simulink model "stimfun"  (R2023a)
settings: Solver=VariableStepAuto  StartTime=0.0  StopTime=10.0  RelTol=1e-3
libraries: simulink x1
settings Model: Creator=s202421  LastModifiedBy=s202421

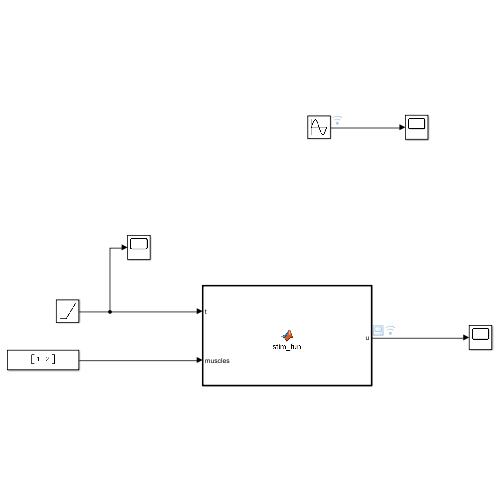
[thumbnail: Simulink's stored preview of the top-level diagram]
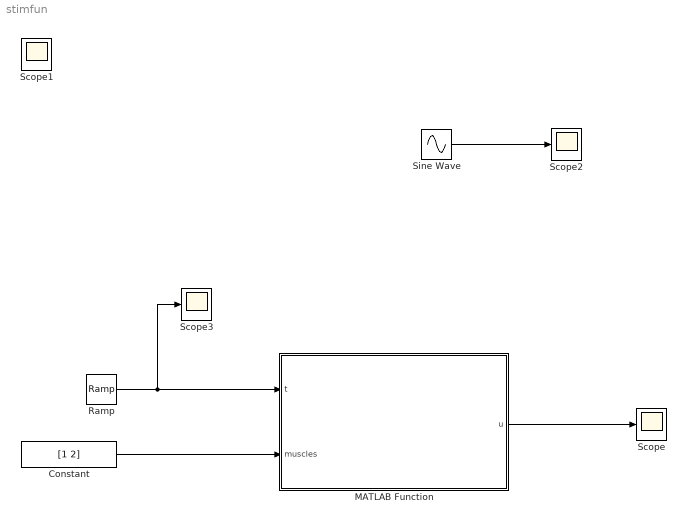
== system stimfun ==
  Constant : Constant  Value=[1 2]  VectorParams1D=off
  MATLAB Function : MATLAB Function  TreatAsAtomicUnit=on
  Ramp : simulink/Sources/Ramp  slope=1  start=0  InitialOutput=0
  Scope{,1..3} (4 alike) : Scope
  Sine Wave : Sin  SampleTime=0
  wires:
  Constant/1 -> MATLAB Function/2(muscles)
  MATLAB Function/1(u) -> Scope/1
  Sine Wave/1 -> Scope2/1
  Ramp/1 -> Scope3/1, MATLAB Function/1(t)

== matlab function stimfun/MATLAB Function ==
  data: t input; u output; muscles input
function u  = stim_fun(t, muscles)
    nmus = 138;
    u = zeros(nmus,1);
    %u = 0;
    if muscles ~= 0
        if t > 2.5
            u(muscles) = 1;
            %u = 1;
        end 
        if t > 5
            u(muscles)=0;
            %u = 0;
        end
    end
end
